simulink model "FunctionCallTest"  (R2020a)
settings: Solver=FixedStepAuto  StartTime=0.0  StopTime=10.0  RelTol=1e-3
libraries: simulink x1
settings Model: Creator=sadamu  LastModifiedBy=sadamu
settings OptimizationCC: DefaultParameterBehavior=Inlined  UseDivisionForNetSlopeComputation=on  GainParamInheritBuiltInType=on  UseFloatMulNetSlope=on  InlineInvariantSignals=on  EfficientFloat2IntCast=on  LifeSpan=1
settings HardwareCC: ProdLongLongMode=on
settings SFSimCC: MATLABDynamicMemAlloc=off
settings RTWCC: GenerateReport=on  LaunchReport=on
settings CodeAppCC: GenerateComments=off
settings GRTTargetCC: CombineSignalStateStructs=on  MatFileLogging=off  SupportVariableSizeSignals=on

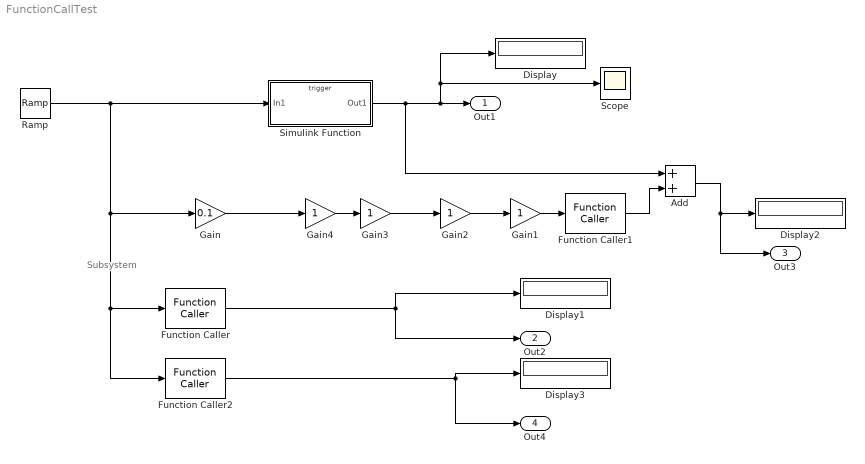
== system FunctionCallTest ==
  note: Subsystem
  Add : Sum
  Display{,1..3} (4 alike) : Display
  Function Caller : FunctionCaller  FunctionPrototype=y = f(u)  InputArgumentSpecifications=<Enter example>  OutputArgumentSpecifications=<Enter example>
  Function Caller1 : FunctionCaller  FunctionPrototype=y = f(u)  InputArgumentSpecifications=<Enter example>  OutputArgumentSpecifications=<Enter example>
  Function Caller2 : FunctionCaller  FunctionPrototype=y = f(u)  InputArgumentSpecifications=<Enter example>  OutputArgumentSpecifications=<Enter example>
  Gain : Gain  Gain=0.1
  Gain{1..4} (4 alike) : Gain
  Ramp : simulink/Sources/Ramp  slope=1  start=0  InitialOutput=0
  Scope : Scope
  Simulink Function : Subsystem  TreatAsAtomicUnit=on
  Out1 : Outport
  Out2 : Outport  Port=2
  Out3 : Outport  Port=3
  Out4 : Outport  Port=4
  wires:
  Simulink Function/1(Out1) -> Add/1, Display/1, Scope/1, Out1/1
  Function Caller1/1 -> Add/2
  Gain/1 -> Gain4/1
  Gain4/1 -> Gain3/1
  Gain3/1 -> Gain2/1
  Gain2/1 -> Gain1/1
  Gain1/1 -> Function Caller1/1
  Function Caller2/1 -> Display3/1, Out4/1
  Function Caller/1 -> Out2/1, Display1/1
  Ramp/1 -> Gain/1, Function Caller2/1, Function Caller/1, Simulink Function/1(In1)
  Add/1 -> Out3/1, Display2/1

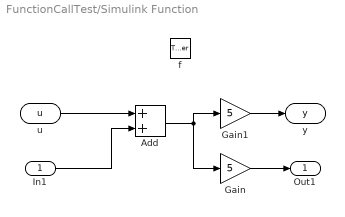
== system FunctionCallTest/Simulink Function ==
  In1 : Inport
  f : TriggerPort  TriggerType=function-call  IsSimulinkFunction=on  FunctionName=f  FunctionVisibility=scoped  VariantControl=(inherit)
  Add : Sum
  Gain : Gain  Gain=5
  Gain1 : Gain  Gain=5
  u : ArgIn  DisableCoverage=on  ArgumentName=u
  y : ArgOut  DisableCoverage=on  ArgumentName=y
  Out1 : Outport
  wires:
  u/1 -> Add/1
  Gain/1 -> Out1/1
  In1/1 -> Add/2
  Gain1/1 -> y/1
  Add/1 -> Gain/1, Gain1/1
